simulink model "lab2"  (R2023b)
settings: Solver=VariableStepAuto  StartTime=0.0  StopTime=10.0  RelTol=1e-3
undefined symbols (not defined in the file or in its folder): DiscIntNeverNeededParam, par, q0, qdot0, torques, wrenches
settings Model: Creator=rpl  LastModifiedBy=rpl

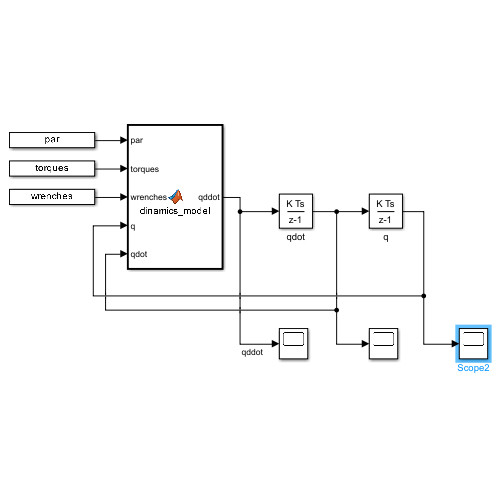
[thumbnail: Simulink's stored preview of the top-level diagram]
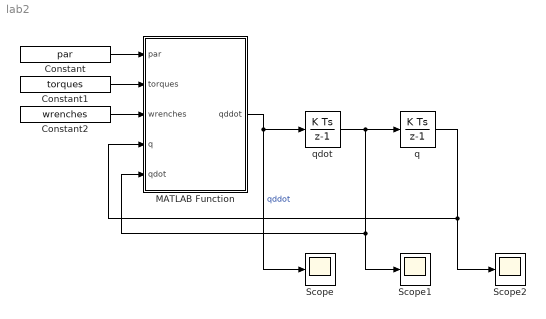
== system lab2 ==
  Constant : Constant  Value=par
  Constant1 : Constant  Value=torques  OutDataTypeStr=double
  Constant2 : Constant  Value=wrenches
  MATLAB Function : MATLAB Function  TreatAsAtomicUnit=on
  Scope : Scope
  Scope1 : Scope
  Scope2 : Scope
  q : DiscreteIntegrator  InitialCondition=q0  SampleTime=0.001  ICPrevOutput=DiscIntNeverNeededParam  ICPrevScaledInput=DiscIntNeverNeededParam
  qdot : DiscreteIntegrator  InitialCondition=qdot0  SampleTime=-1  ICPrevOutput=DiscIntNeverNeededParam  ICPrevScaledInput=DiscIntNeverNeededParam
  wires:
  MATLAB Function/1(qddot) -> Scope/1, qdot/1  "qddot"
  qdot/1 -> Scope1/1, MATLAB Function/5(qdot), q/1
  q/1 -> Scope2/1, MATLAB Function/4(q)
  Constant/1 -> MATLAB Function/1(par)
  Constant1/1 -> MATLAB Function/2(torques)
  Constant2/1 -> MATLAB Function/3(wrenches)

== matlab function lab2/MATLAB Function ==
  data: par input; torques input; wrenches input; q input; qddot output; qdot input
function qddot = dinamics_model(par, torques, wrenches, q, qdot)

    m1 = par(1);
    m2 = par(2);
    l1 = par(3);
    l2 = par(4);
    b1 = par(5);
    b2 = par(6);
    g = par(7);

    % sines and cosines
    sq1 = sin(q(1));
    sq2 = sin(q(2));
    cq1 = cos(q(1));
    cq2 = cos(q(2));
    sq12 = sin(q(1)+q(2));
    cq12 = cos(q(1)+q(2));
    
    % Calculate M(1)
    Msim = m2*(l1*l2*cq2 + l2^2); % simetrical term
    M = [m1*l1^2+m2*(l1^2+2*l1*l2*cq2+l2^2), Msim;
         Msim, m2*l2^2];
         
    % Calculate C(q, qdot)*qdot
    Cqdot = [-m2*l1*l2*sq2*(2*qdot(1)*qdot(2)+qdot(2)^2);
              m2*l1*l2*qdot(1)^2*sq2];

    % Calculate Fb
    Fb = [b1, 0;
          0, b2];

    % Calculate g(q)
    g = [(m1+m2)*l1*g*cq1+m2*g*l2*cq12;
          m2*g*l2*cq12];

    % Calculate J(q)
    J = [-l1*sq1-l2*sq12, -l2*sq12;
          l1*cq1+l2*cq12,  l2*cq12];

    % Calcualte tau_ext
    tau_ext = J' * wrenches;
    
    % Calculate qddot
    qddot = inv(M)*(torques - Cqdot - Fb*qdot - g + tau_ext);
